simulink model "Tim1VariableFreq"  (R2015b)
settings: Solver=FixedStepDiscrete  StartTime=0.0  StopTime=10.0  FixedStep=0.5  RelTol=1e-3
libraries: ADC_Lib x1, STM32_Config_Lib x1, TIMERS_Lib x1
settings Model: Creator=reynaudp  LastModifiedBy=reynaudp
settings DataIOCC: SaveFormat=Array
settings OptimizationCC: ExpressionDepthLimit=2147483647  OptimizeModelRefInitCode=on  LifeSpan=1
settings DebuggingCC: UnderspecifiedInitializationDetection=Classic  MergeDetectMultiDrivingBlocksExec=none  SolverPrmCheckMsg=warning  StateNameClashWarn=warning
settings HardwareCC: ProdBitPerPointer=32  ProdLargestAtomicInteger=Integer  ProdWordSize=32  ProdHWDeviceType=STMicroelectronics->STM32 32-bit Cortex-M
settings RTWCC: SystemTargetFile=stm32.tlc  TemplateMakefile=stm32.tmf  Description=stm32 (Embedded Target)  GenerateReport=on  IncludeHyperlinkInReport=on  LaunchReport=on
settings CodeAppCC: IgnoreCustomStorageClasses=off  MaxIdLength=64  CustomSymbolStrType=$N$R$M  SimulinkBlockComments=off  InternalIdentifier=Classic
settings STFCustomTargetCC: ParMdlRefBuildCompliant=on  ConcurrentExecutionCompliant=off  IncludeMdlTerminateFcn=off  GeneratePreprocessorConditionals=Use local settings  CombineOutputUpdateFcns=on  ERTCustomFileBanners=on  SupportContinuousTime=off  SupportNonInlinedSFcns=off  MATLABClassNameForMDSCustomization=Simulink.SoftwareTarget.ERTCustomization  CPPClassGenCompliant=off  GRTInterface=off  SystemTargetFile=stm32.tlc
settings ERTTargetCC: CompOptLevelCompliant=off  ConcurrentExecutionCompliant=off  IncludeMdlTerminateFcn=off  ERTFirstTimeCompliant=off  ModelStepFunctionPrototypeControlCompliant=off  CPPClassGenCompliant=off  UseToolchainInfoCompliant=off  ERTSrcFileBannerTemplate=sourceFileTemplate.cgt  ERTHdrFileBannerTemplate=sourceFileTemplate.cgt  ERTDataSrcFileTemplate=sourceFileTemplate.cgt  ERTDataHdrFileTemplate=sourceFileTemplate.cgt  ERTCustomFileTemplate=customRoutineProcess.tlc
settings ConfigComp: CovModelRefEnable=Off  CovSFcnEnable=off

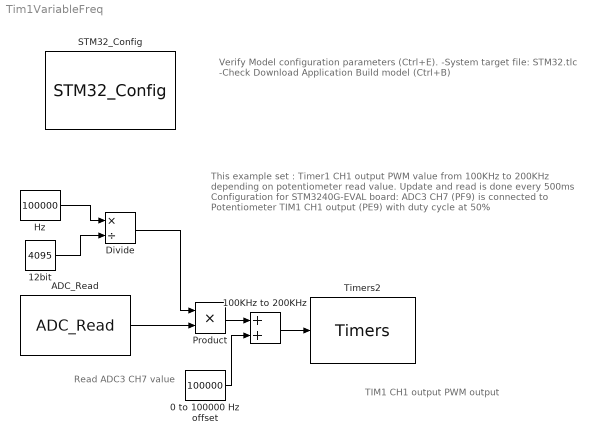
== system Tim1VariableFreq ==
  note: Read ADC3 CH7 value
  note: TIM1 CH1 output
      | PWM output
  note: Verify Model configuration parameters (Ctrl+E).
      | 	-System target file: STM32.tlc
      | 	-Check Download Application
      | Build model (Ctrl+B)
  note: This example set :
      | Timer1 CH1 output PWM value from
      | 100KHz to 200KHz depending on potentiometer read value.
      |
      | Update and read is done every 500ms
      |
      | Configuration for STM3240G-EVAL board:
      | ADC3 CH7 (PF9) is connected to Potentiometer
      | TIM1 CH1 output (PE9) with duty cycle at 50%
  0 to 100000 Hz offset : Constant  Value=100000
  100KHz to 200KHz : Sum
  12bit : Constant  Value=4095  OutDataTypeStr=single
  ADC_Read : ADC_Lib/ADC_Read  ADC_Name=ADC3  ADC_Ch0=off  ADC_Ch1=off  ADC_Ch2=off  ADC_Ch3=off  ADC_Ch4=off  ADC_Ch5=off  ADC_Ch6=off  ADC_Ch7=on  ADC_Ch8=off  ADC_Ch9=off  ADC_Ch10=off  ADC_Ch11=off  ADC_Ch12=off  ADC_Ch13=off  ADC_Ch14=off  ADC_Ch15=off  ADC_Ch16=off  ADC_Ch17=off  ADC_Ch18=off  RgRk1=on  RgRk2=off  RgRk3=off  RgRk4=off  RgRk1_Ch=Ch7_r1  RgRk2_Ch=off  RgRk3_Ch=off  RgRk4_Ch=off  RgRk5=off  RgRk6=off  RgRk7=off  RgRk8=off  RgRk5_Ch=off  RgRk6_Ch=off  RgRk7_Ch=off  RgRk8_Ch=off  RgRk9=off  RgRk10=off  RgRk11=off  RgRk12=off  RgRk9_Ch=off  RgRk10_Ch=off  RgRk11_Ch=off  RgRk12_Ch=off  RgRk13=off  RgRk14=off  RgRk15=off  RgRk16=off  RgRk13_Ch=off  RgRk14_Ch=off  RgRk15_Ch=off  RgRk16_Ch=off  InjRk1=off  InjRk2=off  InjRk3=off  InjRk4=off  InjRk1_Ch=off  InjRk2_Ch=off  InjRk3_Ch=off  InjRk4_Ch=off  ADC_Trig=Not used  ADC_TrigEdge=NONE  DmaReq=off  ItReq=on  AWD_Mode=NOT_USED  AWD_Ch=0  AWD_HThres=0  AWD_LThres=0  AWD_En_Int=off  AWD2_HThres=0  AWD2_LThres=0  AWD2_En_Int=off  AWD3_HThres=0  AWD3_LThres=0  AWD3_En_Int=off  EOC_IT=off  JEOC_IT=off  AWD_IT=off  OVR_IT=off  ADC_RegNb=1  ADC_RegCh0=off  ADC_RegCh1=off  ADC_RegCh2=off  ADC_RegCh3=off  ADC_RegCh4=off  ADC_RegCh5=off  ADC_RegCh6=off  ADC_RegCh7=on  ADC_RegCh8=off  ADC_RegCh9=off  ADC_RegCh10=off  ADC_RegCh11=off  ADC_RegCh12=off  ADC_RegCh13=off  ADC_RegCh14=off  ADC_RegCh15=off  ADC_RegCh16=off  ADC_RegCh17=off  ADC_RegCh18=off  ADC_InjNb=0  ADC_InjCh0=off  ADC_InjCh1=off  ADC_InjCh2=off  ADC_InjCh3=off  ADC_InjCh4=off  ADC_InjCh5=off  ADC_InjCh6=off  ADC_InjCh7=off  ADC_InjCh8=off  ADC_InjCh9=off  ADC_InjCh10=off  ADC_InjCh11=off  ADC_InjCh12=off  ADC_InjCh13=off  ADC_InjCh14=off  ADC_InjCh15=off  ADC_InjCh16=off  ADC_InjCh17=off  ADC_InjCh18=off  ADC_RegRank0=0  ADC_RegRank1=0  ADC_RegRank2=0  ADC_RegRank3=0  ADC_RegRank4=0  ADC_RegRank5=0  ADC_RegRank6=0  ADC_RegRank7=1  ADC_RegRank8=0  ADC_RegRank9=0  ADC_RegRank10=0  ADC_RegRank11=0  ADC_RegRank12=0  ADC_RegRank13=0  ADC_RegRank14=0  ADC_RegRank15=0  ADC_RegRank16=0  ADC_RegRank17=0  ADC_RegRank18=0  ADC_InjRank0=0  ADC_InjRank1=0  ADC_InjRank2=0  ADC_InjRank3=0  ADC_InjRank4=0  ADC_InjRank5=0  ADC_InjRank6=0  ADC_InjRank7=0  ADC_InjRank8=0  ADC_InjRank9=0  ADC_InjRank10=0  ADC_InjRank11=0  ADC_InjRank12=0  ADC_InjRank13=0  ADC_InjRank14=0  ADC_InjRank15=0  ADC_InjRank16=0  ADC_InjRank17=0  ADC_InjRank18=0  NbADC=1  CurrentADC=ADC3
  Divide : Product  Inputs=*/
  Hz : Constant  Value=100000  OutDataTypeStr=single
  Product : Product  RndMeth=Zero
  STM32_Config : STM32_Config_Lib/STM32_Config  Priority=0  Project_Path=.\  Config_File=Tim1VariableFreq.ioc  MCU_Name=STM32F417IGHx
  Timers2 : TIMERS_Lib/Timers  currentTIM=TIM1  TIM_Name=TIM1  TIM_APBClock=84000000  TIM_CKD=1  TIM_Set_Clk=on  TIM_Prescaler=7  TIM_Clock=10500000.00  Variable_frequency=on  TIM_Set_OutFreq=on  TIM_ARR=51  Output_frequency=201923.08  Repetition_counter=0  TIM_Mode=Up  TIM_DMA=none  TIM_IRQ=off  TIM_IRQ_ONLY=off  TIM_UP=off  TIM_TRG=off  TIM_COM=off  TIM_BRK=off  NbTIM=1  CH1_enable=on  CH1N_enable=off  CH1_type=Output_PWM  CH1_DMA=off  CH1_int=off  CH1_edge=Rising  CH1_div=1  CH1_variable_duty=off  CH1_set_pulse=on  CH1_output_duty=50  CH1_pulse=25  CH2_enable=off  CH2N_enable=off  CH2_type=Unknown  CH2_DMA=off  CH2_int=off  CH2_edge=Rising  CH2_div=1  CH2_variable_duty=off  CH2_set_pulse=off  CH2_output_duty=0.00  CH2_pulse=0  CH3_enable=off  CH3N_enable=off  CH3_type=Unknown  CH3_DMA=off  CH3_int=off  CH3_edge=Rising  CH3_div=1  CH3_variable_duty=off  CH3_set_pulse=off  CH3_output_duty=0.00  CH3_pulse=0  CH4_enable=off  CH4N_enable=off  CH4_type=Unknown  CH4_DMA=off  CH4_int=off  CH4_edge=Rising  CH4_div=1  CH4_variable_duty=off  CH4_set_pulse=off  CH4_output_duty=0.00  CH4_pulse=0
  wires:
  Hz/1 -> Divide/1
  ADC_Read/1 -> Product/2
  12bit/1 -> Divide/2
  Divide/1 -> Product/1
  Product/1 -> 100KHz to 200KHz/1
  0 to 100000 Hz offset/1 -> 100KHz to 200KHz/2
  100KHz to 200KHz/1 -> Timers2/1
